simulink model "kalman_filter3"  (Simulink 7.8)
settings: Solver=FixedStepDiscrete  SolverMode=SingleTasking  StartTime=0.0  StopTime=0.02  RelTol=1e-3
values from neighbouring files (symbols this model uses):
  hmusik = fir1(nf-1, 0.4)    [block_lms_.m]
  hr = 0.8.^(0:nf-1)    [block_lms_.m]
  Ts = 1/fs    (= 6.25e-05)    [G722_1.m]    (also in adaptiv_2.m = 0.001; adaptiv_3.m = 0.001; adaptiv_4.m = 0.001; adaptiv_5.m = 0.001)
undefined symbols (not defined in the file or in its folder): get, stoerung
libraries: dspstat3 x2, dspsigops x1, dspobslib x1, dspsrcs4 x1, dspsnks4 x1
settings Model: Creator=svenhoffmann  LastModifiedBy=josef  ExtModeAutoUpdateStatusClock=off
settings DataIOCC: SignalLoggingName=sigsOut
settings DebuggingCC: SaveWithParameterizedLinksMsg=none  SignalResolutionControl=TryResolveAllWithWarning  SolverPrmCheckMsg=none  MultiTaskDSMMsg=warning  MultiTaskCondExecSysMsg=none  StrictBusMsg=None
settings HardwareCC: TargetUnknown=on
settings RTWCC: IncludeERTFirstTime=on

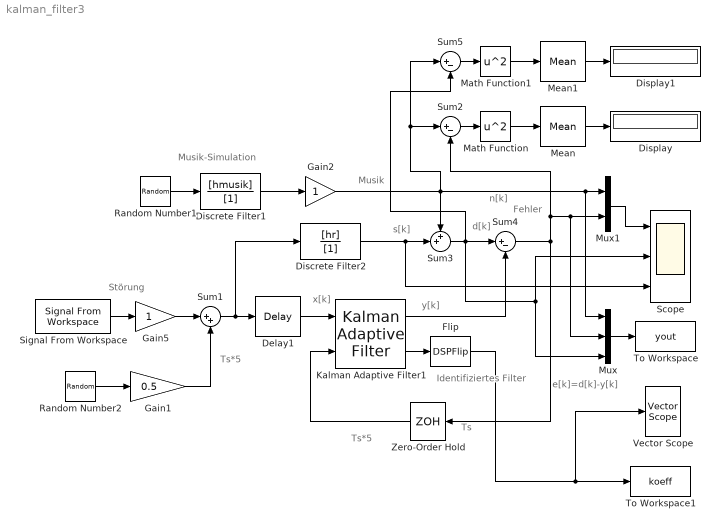
== system kalman_filter3 ==
  note: Musik
  note: Störung
  note: Musik-Simulation
  note: Fehler
  note: s[k]
  note: n[k]
  note: d[k]
  note: y[k]
  note: x[k]
  note: e[k]=d[k]-y[k]
  note: Identifiziertes Filter
  note: Ts*5
  note: Ts
  note: Ts*5
  Delay1 : dspsigops/Delay  InputProcessing=Inherited (this choice will be removed - see release notes)  dly_unit=Samples  delay=3  ic_detail=off  dif_ic_for_ch=off  dif_ic_for_dly=off  ic=0  reset_popup=None
  Discrete Filter1 : DiscreteFilter  Numerator=[hmusik]  Denominator=[1]  SampleTime=Ts
  Discrete Filter2 : DiscreteFilter  Numerator=[hr]  Denominator=[1]  SampleTime=5*Ts
  Display : Display
  Display1 : Display
  Flip : DSPFlip
  Gain1 : Gain  Gain=0.5  SaturateOnIntegerOverflow=on  OutDataTypeStr=Inherit: Same as input  ParamDataTypeStr=Inherit: Same as input
  Gain2 : Gain  SaturateOnIntegerOverflow=on  OutDataTypeStr=Inherit: Same as input  ParamDataTypeStr=Inherit: Same as input
  Gain5 : Gain  SaturateOnIntegerOverflow=on  OutDataTypeStr=Inherit: Same as input  ParamDataTypeStr=Inherit: Same as input
  Kalman Adaptive Filter1 : dspobslib/Kalman Adaptive Filter  Ntaps=M  Jmin=1  q=0  ic0=0  K0=1  Adapt=off  RstPort=None
  Math Function : Math  Operator=square  SaturateOnIntegerOverflow=on
  Math Function1 : Math  Operator=square  SaturateOnIntegerOverflow=on
  Mean : dspstat3/Mean  run=on  reset_popup=None  InputProcessing=Inherited (this choice will be removed - see release notes)  directionMode=Each column  dimension=1  treatSBRowAsCol=on  roiEnable=off  roiType=Rectangles  roiPortion=Entire ROI  roiOutput=Individual statistics for each ROI  roiFlag=off  outputDataTypeStr=Inherit: Same as accumulator  outputLastDataTypeStr=Inherit: Same as accumulator  outputMin=[]  outputMax=[]  roundingMode=Floor  overflowMode=off
  Mean1 : dspstat3/Mean  run=on  reset_popup=None  InputProcessing=Inherited (this choice will be removed - see release notes)  directionMode=Each column  dimension=1  treatSBRowAsCol=on  roiEnable=off  roiType=Rectangles  roiPortion=Entire ROI  roiOutput=Individual statistics for each ROI  roiFlag=off  outputDataTypeStr=Inherit: Same as accumulator  outputLastDataTypeStr=Inherit: Same as accumulator  outputMin=[]  outputMax=[]  roundingMode=Floor  overflowMode=off
  Mux : Mux  Inputs=3
  Mux1 : Mux  Inputs=2
  Random Number1 : RandomNumber  Seed=1739  SampleTime=Ts
  Random Number2 : RandomNumber  SampleTime=Ts*5
  Scope : Scope  NumInputPorts=3
      settings: YMin=-7~-4.5~-3.5  YMax=5~4.5~3.5
  Signal From Workspace : dspsrcs4/Signal From Workspace  X=stoerung(:,1)  Ts=Ts*5  nsamps=1  OutputAfterFinalValue=Setting to zero  ignoreOrWarnInputAndFrameLengths=off
  Sum1 : Sum  Inputs=|++  SaturateOnIntegerOverflow=on
  Sum2 : Sum  Inputs=|+-  SaturateOnIntegerOverflow=on
  Sum3 : Sum  Inputs=++|  SaturateOnIntegerOverflow=on
  Sum4 : Sum  Inputs=|+-  SaturateOnIntegerOverflow=on
  Sum5 : Sum  Inputs=|+-  SaturateOnIntegerOverflow=on
  To Workspace : ToWorkspace  VariableName=yout  SampleTime=-1  SaveFormat=Structure With Time
  To Workspace1 : ToWorkspace  VariableName=koeff  SampleTime=-1  SaveFormat=Structure
      settings: Decimation=100
  Vector Scope : dspsnks4/Vector Scope  ScopeProperties=off  Domain=Time  HorizSpan=1  DisplayProperties=off  AxisGrid=on  Memory=off  FrameNumber=on  AxisLegend=off  AxisZoom=off  OpenScopeAtSimStart=on  OpenScopeImmediately=off  FigPos=get(0,'defaultfigureposition')  AxisProperties=off  XUnits=Hertz  XRange=[0...Fs/2]  InheritXIncr=on  XIncr=1  XLabel=Time  XLimit=Auto  XMin=0  XMax=1  XStart=0  YUnits=dB  YLabel=Amplitude  LineProperties=on  LineMarkers=*  XAxisParamsVer=6.8
      settings: YMin=-0.138141172855862  YMax=1.04495133014087
  Zero-Order Hold : ZeroOrderHold  SampleTime=Ts*5
  wires:
  Discrete Filter2/1 -> Sum3/2, Scope/3
  Sum3/1 -> Mux/3, Scope/2, Sum5/2, Sum4/1
  Sum4/1 -> Sum2/2, Mux/2, Mux1/2, Zero-Order Hold/1
  Random Number1/1 -> Discrete Filter1/1
  Gain2/1 -> Sum3/1, Mux/1, Mux1/1, Sum2/1, Sum5/1
  Discrete Filter1/1 -> Gain2/1
  Sum2/1 -> Math Function/1
  Math Function/1 -> Mean/1
  Mean/1 -> Display/1
  Mux/1 -> To Workspace/1
  Kalman Adaptive Filter1/2 -> Flip/1
  Flip/1 -> Vector Scope/1, To Workspace1/1
  Signal From Workspace/1 -> Gain5/1
  Mux1/1 -> Scope/1
  Gain5/1 -> Sum1/1
  Sum1/1 -> Delay1/1, Discrete Filter2/1
  Random Number2/1 -> Gain1/1
  Gain1/1 -> Sum1/2
  Sum5/1 -> Math Function1/1
  Math Function1/1 -> Mean1/1
  Mean1/1 -> Display1/1
  Delay1/1 -> Kalman Adaptive Filter1/1
  Kalman Adaptive Filter1/1 -> Sum4/2
  Zero-Order Hold/1 -> Kalman Adaptive Filter1/2
